simulink model "downlink_4c2t"  (Simulink 8.7)
settings: Solver=VariableStepDiscrete  StartTime=0.0  StopTime=DUC_LINEUP_param.endTime  RelTol=1e-3
PreLoadFcn:
  | % Run the setup script when the model is opened
  | setup_downlink_4c2t;
InitFcn:
  | % Run the setup script again just before the
  | % model is run, so that any updates made
  | % after opening are applied.
  | setup_downlink_4c2t;
  | 
  | %% DSPBuilder Start
  | alt_dspbuilder_update_model(bdroot)
  | %% DSPBuilder End
values from neighbouring files (symbols this model uses):
  LUTS_DPD_CLIP =     [downlink_4c2t_dpd_clip.mat]
  PulsExtention = 128    [setup_downlink_4c2t.m]
  StartAddress1 = Iter1_Param.BaseAddr + 3200    [setup_downlink_4c2t.m]
  StartAddress2 = StartAddress1+1024    [setup_downlink_4c2t.m]
  win = [w(1:PulsExtention) ones(1,Iter0_Param.pulseLen) w(PulsExtention+1:end)]    [setup_downlink_4c2t.m]
undefined symbols (not defined in the file or in its folder): AdvDSPBChannelOutDisplay, AdvDSPBDMemDisplay, dpoly, dspba_ChannelInVis, dspba_ChannelOutVis, dspba_internal_get_channel_ports, dspba_internal_get_demux_ports, DUC_LINEUP_param, evalAionMaskParam, iq_width, Iter0_Param, latency, primtype, REG, UseDontCare, value
undefined symbols (not defined in the file): cfr0_id, cfr_Params0, cfr_Params1, clock_rate, REG_dut_id_addr
libraries: DSPBAPrim x1438, DSPBAControl x77, DSPBAModelBus x71, DSPBABase x40, downlink_4c2t_foldingcfr_3firs_lib x26, DSPBAUtilities x8, downlink_4c2t_lib x4, downlink_4c2t_cordic_lib x2, downlink_4c2t_dpd_clipper x2, DSPBAFilters x2, DSPBAWaveformSynth x2, downlink_4c2t_lduc_lib x1
(part 11 of 17)

== system downlink_4c2t/DUT/Gain_dpd_input/Subsystem ==
  a : Inport
  v : Inport  Port=2
  c : Inport  Port=3
  dpd1_gain_val : Inport  Port=4
  dpd2_gain_val : Inport  Port=5
  ChannelIn : DSPBAPrim/ChannelIn  primtype=channelin  nInputs=dspba_internal_get_channel_ports(gcb)  nOutputs=dspba_internal_get_channel_ports(gcb)  omode=Inherit via internal rule  otype=sfix(16)  scale=2^-15  rndmethod=Unbiased  factor=1  satmethod=Symmetric  shift_vec=[0 1 2 -1]  value=1  inPortNames=['v'; 'c'; '0'; '1'; '2'; '3'; '4'; '5'; '6'; '7'; '8'; '9'; 'A'; 'B'; 'D'; 'E'; 'F'; 'G'; 'H'; 'I'; 'J'; 'K'; 'L'; 'M'; 'N'; 'O'; 'P'; 'Q'; 'R'; 'S'; 'T'; 'U'; 'W'; 'X'; 'Y'; 'Z']  outPortNames=['v'; 'c'; '0'; '1'; '2'; '3'; '4'; '5'; '6'; '7'; '8'; '9'; 'A'; 'B'; 'D'; 'E'; 'F'; 'G'; 'H'; 'I'; 'J'; 'K'; 'L'; 'M'; 'N'; 'O'; 'P'; 'Q'; 'R'; 'S'; 'T'; 'U'; 'W'; 'X'; 'Y'; 'Z']  dspbaimage=dspba_prim.jpg  text=fprintf('In');  style=Optimised  dataSignals=1  foldingEnabled=off  channels=1  sampleRate=200  packetBeginPresent=off  packetBeginEnabled=off  visibilities=dspba_ChannelInVis(gcb)  latencyCorrection=0  version=20141013
  ChannelOut : DSPBAPrim/ChannelOut  primtype=channelout  nInputs=dspba_internal_get_channel_ports(gcb)  nOutputs=dspba_internal_get_channel_ports(gcb)  omode=Inherit via internal rule  otype=sfix(16)  scale=2^-15  rndmethod=Unbiased  factor=1  satmethod=Symmetric  shift_vec=[0 1 2 -1]  value=1  inPortNames=['v'; 'c'; '0'; '1'; '2'; '3'; '4'; '5'; '6'; '7'; '8'; '9'; 'A'; 'B'; 'D'; 'E'; 'F'; 'G'; 'H'; 'I'; 'J'; 'K'; 'L'; 'M'; 'N'; 'O'; 'P'; 'Q'; 'R'; 'S'; 'T'; 'U'; 'W'; 'X'; 'Y'; 'Z']  outPortNames=['v'; 'c'; '0'; '1'; '2'; '3'; '4'; '5'; '6'; '7'; '8'; '9'; 'A'; 'B'; 'D'; 'E'; 'F'; 'G'; 'H'; 'I'; 'J'; 'K'; 'L'; 'M'; 'N'; 'O'; 'P'; 'Q'; 'R'; 'S'; 'T'; 'U'; 'W'; 'X'; 'Y'; 'Z']  dspbaimage=dspba_prim.jpg  text=fprintf('Out%s', AdvDSPBChannelOutDisplay(latency));  style=Optimised  dataSignals=1  foldingEnabled=off  channels=1  sampleRate=200  packetBeginPresent=off  packetBeginEnabled=off  visibilities=dspba_ChannelOutVis(gcb)  latency=4  latencyCorrection=0  version=20141013
  Demux : Demux
  GPIn1 : DSPBAPrim/GPIn  primtype=gpin  nInputs=evalAionMaskParam(gcb,'value',1)  nOutputs=evalAionMaskParam(gcb,'value',1)  omode=Inherit via internal rule  otype=sfix(16)  scale=2^-15  rndmethod=Unbiased  factor=1  satmethod=Symmetric  shift_vec=[0 1 2 -1]  value=1  inPortNames=[' ' ' ' ' ' ' ' ' ' ' ' ' ' ' ' ' ' ' ' ' ' ' ' ' ' ' ' ' ' ' ' ' ' ' ' ' ' ' ' ' ' ' ' ' ' ' ' ' ' ' ' ' ' ' ' ' ' ' ' ' ' ' ' ' ' ' ' ' ']'  outPortNames=[' ' ' ' ' ' ' ' ' ' ' ' ' ' ' ' ' ' ' ' ' ' ' ' ' ' ' ' ' ' ' ' ' ' ' ' ' ' ' ' ' ' ' ' ' ' ' ' ' ' ' ' ' ' ' ' ' ' ' ' ' ' ' ' ' ' ' ' ' ']'  dspbaimage=dspba_prim.jpg  text=fprintf('GPIn');  style=Optimised  visibilities=1024  latencyCorrection=0  version=20090407
  GPIn2 : DSPBAPrim/GPIn  primtype=gpin  nInputs=evalAionMaskParam(gcb,'value',1)  nOutputs=evalAionMaskParam(gcb,'value',1)  omode=Inherit via internal rule  otype=sfix(16)  scale=2^-15  rndmethod=Unbiased  factor=1  satmethod=Symmetric  shift_vec=[0 1 2 -1]  value=1  inPortNames=[' ' ' ' ' ' ' ' ' ' ' ' ' ' ' ' ' ' ' ' ' ' ' ' ' ' ' ' ' ' ' ' ' ' ' ' ' ' ' ' ' ' ' ' ' ' ' ' ' ' ' ' ' ' ' ' ' ' ' ' ' ' ' ' ' ' ' ' ' ']'  outPortNames=[' ' ' ' ' ' ' ' ' ' ' ' ' ' ' ' ' ' ' ' ' ' ' ' ' ' ' ' ' ' ' ' ' ' ' ' ' ' ' ' ' ' ' ' ' ' ' ' ' ' ' ' ' ' ' ' ' ' ' ' ' ' ' ' ' ' ' ' ' ']'  dspbaimage=dspba_prim.jpg  text=fprintf('GPIn');  style=Optimised  visibilities=1024  latencyCorrection=0  version=20090407
  LocalThreshold : DSPBABase/LocalThreshold  margin=DUC_LINEUP_param.ClockMargin  delayRegOrRAMThresholdBits=-1  MediumDualMemThresholdBits=-1  LargeDualMemThresholdBits=-1  hardMultiplierThresholdLuts=-1  complexMultKaratsuba=off  version=0
  Mult{,1..3} (4 alike) : DSPBAPrim/Mult  primtype=mult  nInputs=2  nOutputs=1  omode=Inherit via internal rule  otype=sfix(16)  scale=2^-15  rndmethod=Unbiased  factor=1  satmethod=Symmetric  shift_vec=[0 1 2 -1]  value=0  inPortNames=[' '; ' ';]  outPortNames=[' ']  dspbaimage=dspba_prim.jpg  text=fprintf('X');  style=Optimised  visibilities=8+2^18+2^19  floatPrecision=float32_m23  floatRounding=correct  advOptions=[]  version=20130115
  Mux : Mux
  SynthesisInfo : DSPBAPrim/SynthesisInfo  primtype=synthinfo  nInputs=0  nOutputs=0  omode=Inherit via internal rule  otype=sfix(16)  scale=2^-15  rndmethod=Truncate  factor=1  satmethod=Symmetric  shift_vec=[0 1 2 -1]  value=99  inPortNames=[' '; ' ';]  outPortNames=[' ']  dspbaimage=dspba_prim_ctrl.jpg  text=fprintf('Style=%s', style);  style=Scheduled  visibilities=2^15+2^17+2^18+2^19  constraintInUse=off  constraintRelation=>  constraintLimit=8  bitAccurate=off  version=20150220
  gain_v_out : Outport
  gain_c_out : Outport  Port=2
  gain_real_out : Outport  Port=3
  wires:
  GPIn1/1 -> Mult1/2, Mult/2
  ChannelOut/2 -> gain_c_out/1
  ChannelOut/1 -> gain_v_out/1
  dpd2_gain_val/1 -> GPIn2/1
  dpd1_gain_val/1 -> GPIn1/1
  ChannelOut/3 -> gain_real_out/1
  v/1 -> ChannelIn/1
  c/1 -> ChannelIn/2
  a/1 -> ChannelIn/3
  ChannelIn/1 -> ChannelOut/1
  ChannelIn/2 -> ChannelOut/2
  ChannelIn/3 -> Demux/1
  Demux/1 -> Mult/1
  Demux/2 -> Mult1/1
  Demux/3 -> Mult2/1
  GPIn2/1 -> Mult3/2, Mult2/2
  Demux/4 -> Mult3/1
  Mult/1 -> Mux/1
  Mult1/1 -> Mux/2
  Mult2/1 -> Mux/3
  Mult3/1 -> Mux/4
  Mux/1 -> ChannelOut/3

== system downlink_4c2t/DUT/Gain_duc_input/gain ==
  a : Inport
  v : Inport  Port=2
  c : Inport  Port=3
  carr1_gain_val : Inport  Port=4
  carr2_gain_val : Inport  Port=5
  carr3_gain_val : Inport  Port=6
  carr4_gain_val : Inport  Port=7
  carr5_gain_val : Inport  Port=8
  carr6_gain_val : Inport  Port=9
  carr7_gain_val : Inport  Port=10
  carr8_gain_val : Inport  Port=11
  BitExtract : DSPBAPrim/BitExtract  primtype=bitextract  nInputs=1  nOutputs=1  omode=Specify via dialog  otype=ufix(4)  scale=2^-0  rndmethod=Unbiased  factor=1  satmethod=Symmetric  shift_vec=[0 1 2 -1]  value=1  inPortNames=[' '; ' ';]  outPortNames=[' ']  dspbaimage=dspba_prim.jpg  text=fprintf('..%d', value);  style=Optimised  visibilities=8+1024  version=20090407
  ChannelIn : DSPBAPrim/ChannelIn  primtype=channelin  nInputs=dspba_internal_get_channel_ports(gcb)  nOutputs=dspba_internal_get_channel_ports(gcb)  omode=Inherit via internal rule  otype=sfix(16)  scale=2^-15  rndmethod=Unbiased  factor=1  satmethod=Symmetric  shift_vec=[0 1 2 -1]  value=1  inPortNames=['v'; 'c'; '0'; '1'; '2'; '3'; '4'; '5'; '6'; '7'; '8'; '9'; 'A'; 'B'; 'D'; 'E'; 'F'; 'G'; 'H'; 'I'; 'J'; 'K'; 'L'; 'M'; 'N'; 'O'; 'P'; 'Q'; 'R'; 'S'; 'T'; 'U'; 'W'; 'X'; 'Y'; 'Z']  outPortNames=['v'; 'c'; '0'; '1'; '2'; '3'; '4'; '5'; '6'; '7'; '8'; '9'; 'A'; 'B'; 'D'; 'E'; 'F'; 'G'; 'H'; 'I'; 'J'; 'K'; 'L'; 'M'; 'N'; 'O'; 'P'; 'Q'; 'R'; 'S'; 'T'; 'U'; 'W'; 'X'; 'Y'; 'Z']  dspbaimage=dspba_prim.jpg  text=fprintf('In');  style=Optimised  dataSignals=1  foldingEnabled=off  channels=1  sampleRate=200  packetBeginPresent=off  packetBeginEnabled=off  visibilities=dspba_ChannelInVis(gcb)  latencyCorrection=0  version=20141013
  ChannelOut : DSPBAPrim/ChannelOut  primtype=channelout  nInputs=dspba_internal_get_channel_ports(gcb)  nOutputs=dspba_internal_get_channel_ports(gcb)  omode=Inherit via internal rule  otype=sfix(16)  scale=2^-15  rndmethod=Unbiased  factor=1  satmethod=Symmetric  shift_vec=[0 1 2 -1]  value=1  inPortNames=['v'; 'c'; '0'; '1'; '2'; '3'; '4'; '5'; '6'; '7'; '8'; '9'; 'A'; 'B'; 'D'; 'E'; 'F'; 'G'; 'H'; 'I'; 'J'; 'K'; 'L'; 'M'; 'N'; 'O'; 'P'; 'Q'; 'R'; 'S'; 'T'; 'U'; 'W'; 'X'; 'Y'; 'Z']  outPortNames=['v'; 'c'; '0'; '1'; '2'; '3'; '4'; '5'; '6'; '7'; '8'; '9'; 'A'; 'B'; 'D'; 'E'; 'F'; 'G'; 'H'; 'I'; 'J'; 'K'; 'L'; 'M'; 'N'; 'O'; 'P'; 'Q'; 'R'; 'S'; 'T'; 'U'; 'W'; 'X'; 'Y'; 'Z']  dspbaimage=dspba_prim.jpg  text=fprintf('Out%s', AdvDSPBChannelOutDisplay(latency));  style=Optimised  dataSignals=1  foldingEnabled=off  channels=1  sampleRate=200  packetBeginPresent=off  packetBeginEnabled=off  visibilities=dspba_ChannelOutVis(gcb)  latency=5  latencyCorrection=0  version=20141013
  GPIn{1..8} (8 alike) : DSPBAPrim/GPIn  primtype=gpin  nInputs=evalAionMaskParam(gcb,'value',1)  nOutputs=evalAionMaskParam(gcb,'value',1)  omode=Inherit via internal rule  otype=sfix(16)  scale=2^-15  rndmethod=Unbiased  factor=1  satmethod=Symmetric  shift_vec=[0 1 2 -1]  value=1  inPortNames=[' ' ' ' ' ' ' ' ' ' ' ' ' ' ' ' ' ' ' ' ' ' ' ' ' ' ' ' ' ' ' ' ' ' ' ' ' ' ' ' ' ' ' ' ' ' ' ' ' ' ' ' ' ' ' ' ' ' ' ' ' ' ' ' ' ' ' ' ' ']'  outPortNames=[' ' ' ' ' ' ' ' ' ' ' ' ' ' ' ' ' ' ' ' ' ' ' ' ' ' ' ' ' ' ' ' ' ' ' ' ' ' ' ' ' ' ' ' ' ' ' ' ' ' ' ' ' ' ' ' ' ' ' ' ' ' ' ' ' ' ' ' ' ']'  dspbaimage=dspba_prim.jpg  text=fprintf('GPIn');  style=Optimised  visibilities=1024  latencyCorrection=0  version=20090407
  LocalThreshold : DSPBABase/LocalThreshold  margin=DUC_LINEUP_param.ClockMargin  delayRegOrRAMThresholdBits=-1  MediumDualMemThresholdBits=-1  LargeDualMemThresholdBits=-1  hardMultiplierThresholdLuts=-1  complexMultKaratsuba=off  version=0
  Mult : DSPBAPrim/Mult  primtype=mult  nInputs=2  nOutputs=1  omode=Inherit via internal rule  otype=sfix(16)  scale=2^-15  rndmethod=Unbiased  factor=1  satmethod=Symmetric  shift_vec=[0 1 2 -1]  value=0  inPortNames=[' '; ' ';]  outPortNames=[' ']  dspbaimage=dspba_prim.jpg  text=fprintf('X');  style=Optimised  visibilities=8+2^18+2^19  floatPrecision=float32_m23  floatRounding=correct  advOptions=[]  version=20130115
  Mux : DSPBAPrim/Mux  primtype=mux  nInputs=evalAionMaskParam(gcb,'value',1)+1  nOutputs=1  omode=Inherit via internal rule  otype=sfix(16)  scale=2^-15  rndmethod=Unbiased  factor=1  satmethod=Symmetric  shift_vec=[0 1 2 -1]  value=8  inPortNames=['s '; 'd0'; 'd1'; 'd2'; 'd3'; 'd4'; 'd5'; 'd6'; 'd7'; 'd8'; 'd9';]  outPortNames=[' ']  dspbaimage=dspba_prim.jpg  text=fprintf('%s', primtype);  style=Optimised  visibilities=1032  version=20131025
  SynthesisInfo : DSPBAPrim/SynthesisInfo  primtype=synthinfo  nInputs=0  nOutputs=0  omode=Inherit via internal rule  otype=sfix(16)  scale=2^-15  rndmethod=Truncate  factor=1  satmethod=Symmetric  shift_vec=[0 1 2 -1]  value=99  inPortNames=[' '; ' ';]  outPortNames=[' ']  dspbaimage=dspba_prim_ctrl.jpg  text=fprintf('Style=%s', style);  style=Scheduled  visibilities=2^15+2^17+2^18+2^19  constraintInUse=off  constraintRelation=>  constraintLimit=8  bitAccurate=off  version=20150220
  gain_v_out : Outport
  gain_c_out : Outport  Port=2
  gain_real_out : Outport  Port=3
  wires:
  carr3_gain_val/1 -> GPIn3/1
  BitExtract/1 -> Mux/1
  Mult/1 -> ChannelOut/3
  ChannelIn/2 -> ChannelOut/2, BitExtract/1
  ChannelIn/1 -> ChannelOut/1
  a/1 -> ChannelIn/3
  c/1 -> ChannelIn/2
  v/1 -> ChannelIn/1
  Mux/1 -> Mult/2
  ChannelOut/3 -> gain_real_out/1
  carr8_gain_val/1 -> GPIn8/1
  carr1_gain_val/1 -> GPIn1/1
  carr4_gain_val/1 -> GPIn4/1
  carr5_gain_val/1 -> GPIn5/1
  carr6_gain_val/1 -> GPIn6/1
  carr2_gain_val/1 -> GPIn2/1
  carr7_gain_val/1 -> GPIn7/1
  ChannelIn/3 -> Mult/1
  ChannelOut/1 -> gain_v_out/1
  ChannelOut/2 -> gain_c_out/1
  GPIn1/1 -> Mux/2
  GPIn2/1 -> Mux/3
  GPIn3/1 -> Mux/4
  GPIn4/1 -> Mux/5
  GPIn5/1 -> Mux/6
  GPIn6/1 -> Mux/7
  GPIn7/1 -> Mux/8
  GPIn8/1 -> Mux/9

== system downlink_4c2t/DUT/Gain_summer/Subsystem ==
  a : Inport
  v : Inport  Port=2
  c : Inport  Port=3
  ant1_gain_val : Inport  Port=4
  ant2_gain_val : Inport  Port=5
  BitExtract : DSPBAPrim/BitExtract  primtype=bitextract  nInputs=1  nOutputs=1  omode=Specify via dialog  otype=ufix(4)  scale=2^-0  rndmethod=Unbiased  factor=1  satmethod=Symmetric  shift_vec=[0 1 2 -1]  value=1  inPortNames=[' '; ' ';]  outPortNames=[' ']  dspbaimage=dspba_prim.jpg  text=fprintf('..%d', value);  style=Optimised  visibilities=8+1024  version=20090407
  ChannelIn : DSPBAPrim/ChannelIn  primtype=channelin  nInputs=dspba_internal_get_channel_ports(gcb)  nOutputs=dspba_internal_get_channel_ports(gcb)  omode=Inherit via internal rule  otype=sfix(16)  scale=2^-15  rndmethod=Unbiased  factor=1  satmethod=Symmetric  shift_vec=[0 1 2 -1]  value=1  inPortNames=['v'; 'c'; '0'; '1'; '2'; '3'; '4'; '5'; '6'; '7'; '8'; '9'; 'A'; 'B'; 'D'; 'E'; 'F'; 'G'; 'H'; 'I'; 'J'; 'K'; 'L'; 'M'; 'N'; 'O'; 'P'; 'Q'; 'R'; 'S'; 'T'; 'U'; 'W'; 'X'; 'Y'; 'Z']  outPortNames=['v'; 'c'; '0'; '1'; '2'; '3'; '4'; '5'; '6'; '7'; '8'; '9'; 'A'; 'B'; 'D'; 'E'; 'F'; 'G'; 'H'; 'I'; 'J'; 'K'; 'L'; 'M'; 'N'; 'O'; 'P'; 'Q'; 'R'; 'S'; 'T'; 'U'; 'W'; 'X'; 'Y'; 'Z']  dspbaimage=dspba_prim.jpg  text=fprintf('In');  style=Optimised  dataSignals=1  foldingEnabled=off  channels=1  sampleRate=200  packetBeginPresent=off  packetBeginEnabled=off  visibilities=dspba_ChannelInVis(gcb)  latencyCorrection=0  version=20141013
  ChannelOut : DSPBAPrim/ChannelOut  primtype=channelout  nInputs=dspba_internal_get_channel_ports(gcb)  nOutputs=dspba_internal_get_channel_ports(gcb)  omode=Inherit via internal rule  otype=sfix(16)  scale=2^-15  rndmethod=Unbiased  factor=1  satmethod=Symmetric  shift_vec=[0 1 2 -1]  value=1  inPortNames=['v'; 'c'; '0'; '1'; '2'; '3'; '4'; '5'; '6'; '7'; '8'; '9'; 'A'; 'B'; 'D'; 'E'; 'F'; 'G'; 'H'; 'I'; 'J'; 'K'; 'L'; 'M'; 'N'; 'O'; 'P'; 'Q'; 'R'; 'S'; 'T'; 'U'; 'W'; 'X'; 'Y'; 'Z']  outPortNames=['v'; 'c'; '0'; '1'; '2'; '3'; '4'; '5'; '6'; '7'; '8'; '9'; 'A'; 'B'; 'D'; 'E'; 'F'; 'G'; 'H'; 'I'; 'J'; 'K'; 'L'; 'M'; 'N'; 'O'; 'P'; 'Q'; 'R'; 'S'; 'T'; 'U'; 'W'; 'X'; 'Y'; 'Z']  dspbaimage=dspba_prim.jpg  text=fprintf('Out%s', AdvDSPBChannelOutDisplay(latency));  style=Optimised  dataSignals=1  foldingEnabled=off  channels=1  sampleRate=200  packetBeginPresent=off  packetBeginEnabled=off  visibilities=dspba_ChannelOutVis(gcb)  latency=4  latencyCorrection=0  version=20141013
  GPIn1 : DSPBAPrim/GPIn  primtype=gpin  nInputs=evalAionMaskParam(gcb,'value',1)  nOutputs=evalAionMaskParam(gcb,'value',1)  omode=Inherit via internal rule  otype=sfix(16)  scale=2^-15  rndmethod=Unbiased  factor=1  satmethod=Symmetric  shift_vec=[0 1 2 -1]  value=1  inPortNames=[' ' ' ' ' ' ' ' ' ' ' ' ' ' ' ' ' ' ' ' ' ' ' ' ' ' ' ' ' ' ' ' ' ' ' ' ' ' ' ' ' ' ' ' ' ' ' ' ' ' ' ' ' ' ' ' ' ' ' ' ' ' ' ' ' ' ' ' ' ']'  outPortNames=[' ' ' ' ' ' ' ' ' ' ' ' ' ' ' ' ' ' ' ' ' ' ' ' ' ' ' ' ' ' ' ' ' ' ' ' ' ' ' ' ' ' ' ' ' ' ' ' ' ' ' ' ' ' ' ' ' ' ' ' ' ' ' ' ' ' ' ' ' ']'  dspbaimage=dspba_prim.jpg  text=fprintf('GPIn');  style=Optimised  visibilities=1024  latencyCorrection=0  version=20090407
  GPIn2 : DSPBAPrim/GPIn  primtype=gpin  nInputs=evalAionMaskParam(gcb,'value',1)  nOutputs=evalAionMaskParam(gcb,'value',1)  omode=Inherit via internal rule  otype=sfix(16)  scale=2^-15  rndmethod=Unbiased  factor=1  satmethod=Symmetric  shift_vec=[0 1 2 -1]  value=1  inPortNames=[' ' ' ' ' ' ' ' ' ' ' ' ' ' ' ' ' ' ' ' ' ' ' ' ' ' ' ' ' ' ' ' ' ' ' ' ' ' ' ' ' ' ' ' ' ' ' ' ' ' ' ' ' ' ' ' ' ' ' ' ' ' ' ' ' ' ' ' ' ']'  outPortNames=[' ' ' ' ' ' ' ' ' ' ' ' ' ' ' ' ' ' ' ' ' ' ' ' ' ' ' ' ' ' ' ' ' ' ' ' ' ' ' ' ' ' ' ' ' ' ' ' ' ' ' ' ' ' ' ' ' ' ' ' ' ' ' ' ' ' ' ' ' ']'  dspbaimage=dspba_prim.jpg  text=fprintf('GPIn');  style=Optimised  visibilities=1024  latencyCorrection=0  version=20090407
  LocalThreshold : DSPBABase/LocalThreshold  margin=DUC_LINEUP_param.ClockMargin  delayRegOrRAMThresholdBits=-1  MediumDualMemThresholdBits=-1  LargeDualMemThresholdBits=-1  hardMultiplierThresholdLuts=-1  complexMultKaratsuba=off  version=0
  Mult : DSPBAPrim/Mult  primtype=mult  nInputs=2  nOutputs=1  omode=Inherit via internal rule  otype=sfix(16)  scale=2^-15  rndmethod=Unbiased  factor=1  satmethod=Symmetric  shift_vec=[0 1 2 -1]  value=0  inPortNames=[' '; ' ';]  outPortNames=[' ']  dspbaimage=dspba_prim.jpg  text=fprintf('X');  style=Optimised  visibilities=8+2^18+2^19  floatPrecision=float32_m23  floatRounding=correct  advOptions=[]  version=20130115
  Mux : DSPBAPrim/Mux  primtype=mux  nInputs=evalAionMaskParam(gcb,'value',1)+1  nOutputs=1  omode=Inherit via internal rule  otype=sfix(16)  scale=2^-15  rndmethod=Unbiased  factor=1  satmethod=Symmetric  shift_vec=[0 1 2 -1]  value=2  inPortNames=['s '; 'd0'; 'd1'; 'd2'; 'd3'; 'd4'; 'd5'; 'd6'; 'd7'; 'd8'; 'd9';]  outPortNames=[' ']  dspbaimage=dspba_prim.jpg  text=fprintf('%s', primtype);  style=Optimised  visibilities=1032  version=20131025
  SynthesisInfo : DSPBAPrim/SynthesisInfo  primtype=synthinfo  nInputs=0  nOutputs=0  omode=Inherit via internal rule  otype=sfix(16)  scale=2^-15  rndmethod=Truncate  factor=1  satmethod=Symmetric  shift_vec=[0 1 2 -1]  value=99  inPortNames=[' '; ' ';]  outPortNames=[' ']  dspbaimage=dspba_prim_ctrl.jpg  text=fprintf('Style=%s', style);  style=Scheduled  visibilities=2^15+2^17+2^18+2^19  constraintInUse=off  constraintRelation=>  constraintLimit=6  bitAccurate=off  version=20150220
  gain_v_out : Outport
  gain_c_out : Outport  Port=2
  gain_real_out : Outport  Port=3
  wires:
  GPIn2/1 -> Mux/3
  GPIn1/1 -> Mux/2
  ChannelOut/2 -> gain_c_out/1
  ChannelOut/1 -> gain_v_out/1
  ChannelIn/3 -> Mult/1
  ant2_gain_val/1 -> GPIn2/1
  ant1_gain_val/1 -> GPIn1/1
  ChannelOut/3 -> gain_real_out/1
  Mux/1 -> Mult/2
  v/1 -> ChannelIn/1
  c/1 -> ChannelIn/2
  a/1 -> ChannelIn/3
  ChannelIn/1 -> ChannelOut/1
  ChannelIn/2 -> ChannelOut/2, BitExtract/1
  Mult/1 -> ChannelOut/3
  BitExtract/1 -> Mux/1

== system downlink_4c2t/DUT/LDUC/Mixer_Summer ==
  In_a : Inport
  In_V : Inport  Port=2
  In_C : Inport  Port=3
  In_sync_pulse : Inport  Port=4
  sum_shift : Inport  Port=5
  COMPLEX_MIXER : Subsystem
  PipeReg_2in : downlink_4c2t_foldingcfr_3firs_lib/PipeReg_2in  NPipe=2  Clock_Margin=DUC_LINEUP_param.ClockMargin
      link override ChannelOut: value=2  packetBeginEnabled=off  latency=2
  PipeReg_2in1 : downlink_4c2t_foldingcfr_3firs_lib/PipeReg_2in  NPipe=2  Clock_Margin=DUC_LINEUP_param.ClockMargin
      link override ChannelOut: value=2  packetBeginEnabled=off  latency=2
  SUMMER : Subsystem
  Out_q : Outport
  Out_V : Outport  Port=2
  Out_C : Outport  Port=3
  wires:
  SUMMER/2(q_v) -> Out_V/1
  In_V/1 -> COMPLEX_MIXER/2(v)
  In_C/1 -> COMPLEX_MIXER/3(c)
  SUMMER/1(q) -> Out_q/1
  In_a/1 -> COMPLEX_MIXER/1(a)
  SUMMER/3(q_c) -> Out_C/1
  In_sync_pulse/1 -> COMPLEX_MIXER/4(sync_pulse)
  COMPLEX_MIXER/1(out_I) -> PipeReg_2in/1
  COMPLEX_MIXER/2(out_q) -> PipeReg_2in/2
  COMPLEX_MIXER/4(q_c) -> PipeReg_2in/4
  COMPLEX_MIXER/3(q_v) -> PipeReg_2in/3
  PipeReg_2in/4 -> PipeReg_2in1/4
  PipeReg_2in/1 -> PipeReg_2in1/1
  PipeReg_2in/2 -> PipeReg_2in1/2
  PipeReg_2in/3 -> PipeReg_2in1/3
  PipeReg_2in1/1 -> SUMMER/1(a)
  PipeReg_2in1/2 -> SUMMER/2(a1)
  PipeReg_2in1/3 -> SUMMER/3(v)
  PipeReg_2in1/4 -> SUMMER/4(c)
  sum_shift/1 -> SUMMER/5(sum_shift)

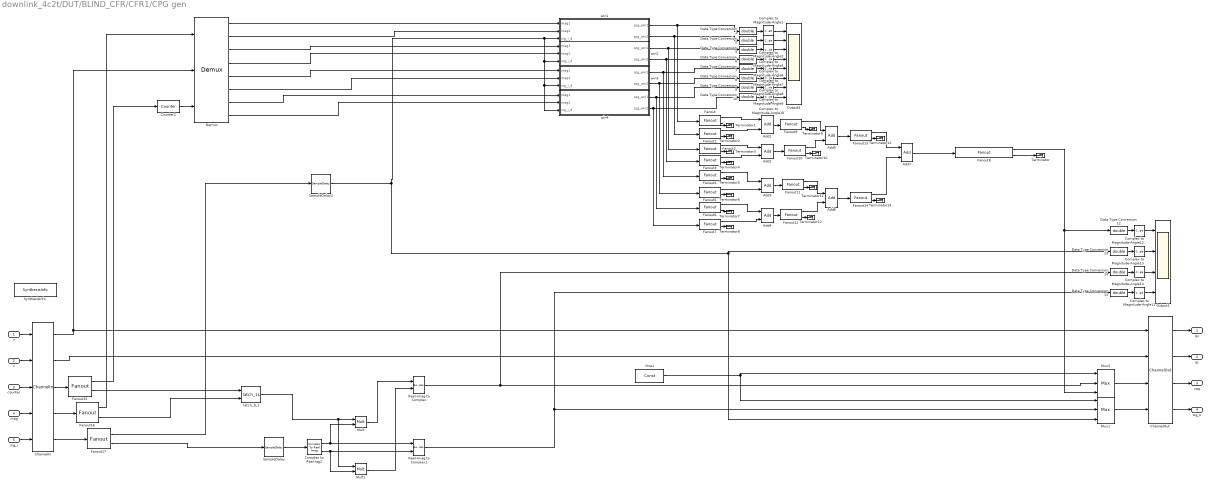
== system downlink_4c2t/DUT/BLIND_CFR/CFR1/CPG gen ==
  v : Inport
  c : Inport  Port=2
  counter : Inport  Port=3
  mag : Inport  Port=4
  sig_i : Inport  Port=5
  Add{1..7} (7 alike) : DSPBAPrim/Add  primtype=add  nInputs=evalAionMaskParam(gcb,'value',1)  nOutputs=1  omode=Inherit via internal rule with word growth  otype=sfix(16)  scale=2^-15  rndmethod=Unbiased  factor=1  satmethod=Symmetric  shift_vec=[0 1 2 -1]  value=2  inPortNames=[' '; ' ';]  outPortNames=[' ']  dspbaimage=dspba_prim.jpg  text=fprintf('+');  style=Optimised  visibilities=1032+2^17+2^18+2^19  genFPC=off  floatRounding=correct  advOptions=[]  version=20130821
  ChannelIn : DSPBAPrim/ChannelIn  primtype=channelin  nInputs=dspba_internal_get_channel_ports(gcb)  nOutputs=dspba_internal_get_channel_ports(gcb)  omode=Inherit via internal rule  otype=sfix(16)  scale=2^-15  rndmethod=Unbiased  factor=1  satmethod=Symmetric  shift_vec=[0 1 2 -1]  value=3  inPortNames=['v'; 'c'; '0'; '1'; '2'; '3'; '4'; '5'; '6'; '7'; '8'; '9'; 'A'; 'B'; 'D'; 'E'; 'F'; 'G'; 'H'; 'I'; 'J'; 'K'; 'L'; 'M'; 'N'; 'O'; 'P'; 'Q'; 'R'; 'S'; 'T'; 'U'; 'W'; 'X'; 'Y'; 'Z']  outPortNames=['v'; 'c'; '0'; '1'; '2'; '3'; '4'; '5'; '6'; '7'; '8'; '9'; 'A'; 'B'; 'D'; 'E'; 'F'; 'G'; 'H'; 'I'; 'J'; 'K'; 'L'; 'M'; 'N'; 'O'; 'P'; 'Q'; 'R'; 'S'; 'T'; 'U'; 'W'; 'X'; 'Y'; 'Z']  dspbaimage=dspba_prim.jpg  text=fprintf('In');  style=Optimised  dataSignals=3  foldingEnabled=off  channels=1  sampleRate=200  packetBeginPresent=off  packetBeginEnabled=off  visibilities=dspba_ChannelInVis(gcb)  latencyCorrection=0  version=20141013
  ChannelOut : DSPBAPrim/ChannelOut  primtype=channelout  nInputs=dspba_internal_get_channel_ports(gcb)  nOutputs=dspba_internal_get_channel_ports(gcb)  omode=Inherit via internal rule  otype=sfix(16)  scale=2^-15  rndmethod=Unbiased  factor=1  satmethod=Symmetric  shift_vec=[0 1 2 -1]  value=2  inPortNames=['v'; 'c'; '0'; '1'; '2'; '3'; '4'; '5'; '6'; '7'; '8'; '9'; 'A'; 'B'; 'D'; 'E'; 'F'; 'G'; 'H'; 'I'; 'J'; 'K'; 'L'; 'M'; 'N'; 'O'; 'P'; 'Q'; 'R'; 'S'; 'T'; 'U'; 'W'; 'X'; 'Y'; 'Z']  outPortNames=['v'; 'c'; '0'; '1'; '2'; '3'; '4'; '5'; '6'; '7'; '8'; '9'; 'A'; 'B'; 'D'; 'E'; 'F'; 'G'; 'H'; 'I'; 'J'; 'K'; 'L'; 'M'; 'N'; 'O'; 'P'; 'Q'; 'R'; 'S'; 'T'; 'U'; 'W'; 'X'; 'Y'; 'Z']  dspbaimage=dspba_prim.jpg  text=fprintf('Out%s', AdvDSPBChannelOutDisplay(latency));  style=Optimised  dataSignals=2  foldingEnabled=off  channels=1  sampleRate=200  packetBeginPresent=off  packetBeginEnabled=off  visibilities=dspba_ChannelOutVis(gcb)  latency=28  latencyCorrection=0  version=20141013
  Complex to Magnitude-Angle{1..2,5..14} (12 alike) : ComplexToMagnitudeAngle  Output=Magnitude
  Complex to Real-Iag2 : ComplexToRealImag
  Counter2 : DSPBAPrim/Counter  primtype=counter  nInputs=1  nOutputs=1  omode=Inherit via internal rule  otype=ufix(16)  scale=2^-0  rndmethod=Unbiased  factor=1  satmethod=Symmetric  shift_vec=[0 1 2 -1]  value=[0 8 1]  inPortNames=[' '; ' ';]  outPortNames=[' ']  dspbaimage=dspba_prim.jpg  text=fprintf('counter\n[%d %d %d]', value(1), value(2), value(3));  style=Optimised  visibilities=8 + 1024  version=20090407
  Data Type Conversion{1..3,6..14} (12 alike) : DataTypeConversion  OutDataTypeStr=double
  Demux : DSPBAPrim/Demux  primtype=demux  nInputs=3  nOutputs=dspba_internal_get_demux_ports(gcb)  omode=Inherit via internal rule  otype=sfix(16)  scale=2^-15  rndmethod=Unbiased  factor=1  satmethod=Symmetric  shift_vec=[0 1 2 3 4 5 6 7]  value=8  inPortNames=['q'; 'v'; 'c']  outPortNames=['c0'; 'c1']  dspbaimage=dspba_prim.jpg  text=fprintf('demux');  style=Optimised  visibilities=1536  version=20100120
  Fanout{,1..17} (18 alike) : DSPBAPrim/Fanout  primtype=fanout  nInputs=1  nOutputs=evalAionMaskParam(gcb,'value',1)  omode=Inherit via internal rule  otype=sfix(16)  scale=2^-15  rndmethod=Unbiased  factor=1  satmethod=Symmetric  shift_vec=[0 1 2 -1]  value=2  inPortNames=[' '; ' ';]  outPortNames=[' ']  dspbaimage=dspba_prim.jpg  text=fprintf('fanout')  style=Optimised  visibilities=2^10+2^18  version=20150501  uninit=off
  Mult : DSPBAPrim/Mult  primtype=mult  nInputs=2  nOutputs=1  omode=Inherit via internal rule  otype=sfix(16)  scale=2^-15  rndmethod=Unbiased  factor=1  satmethod=Symmetric  shift_vec=[0 1 2 -1]  value=0  inPortNames=[' '; ' ';]  outPortNames=[' ']  dspbaimage=dspba_prim.jpg  text=fprintf('X');  style=Optimised  visibilities=8+2^18+2^19  floatPrecision=float32_m23  floatRounding=correct  advOptions=[]  version=20130115
  Mult1 : DSPBAPrim/Mult  primtype=mult  nInputs=2  nOutputs=1  omode=Inherit via internal rule  otype=sfix(16)  scale=2^-15  rndmethod=Unbiased  factor=1  satmethod=Symmetric  shift_vec=[0 1 2 -1]  value=0  inPortNames=[' '; ' ';]  outPortNames=[' ']  dspbaimage=dspba_prim.jpg  text=fprintf('X');  style=Optimised  visibilities=8+2^18+2^19  floatPrecision=float32_m23  floatRounding=correct  advOptions=[]  version=20130115
  Mux1 : DSPBAPrim/Mux  primtype=mux  nInputs=evalAionMaskParam(gcb,'value',1)+1  nOutputs=1  omode=Inherit via internal rule  otype=sfix(16)  scale=2^-15  rndmethod=Unbiased  factor=1  satmethod=Symmetric  shift_vec=[0 1 2 -1]  value=2  inPortNames=['s'; 'd0'; 'd1'; 'd2'; 'd3'; 'd4'; 'd5'; 'd6'; 'd7'; 'd8'; 'd9';]  outPortNames=[' ']  dspbaimage=dspba_prim.jpg  text=fprintf('%s', primtype);  style=Optimised  visibilities=1032  version=20131025
  Mux3 : DSPBAPrim/Mux  primtype=mux  nInputs=evalAionMaskParam(gcb,'value',1)+1  nOutputs=1  omode=Inherit via internal rule  otype=sfix(16)  scale=2^-15  rndmethod=Unbiased  factor=1  satmethod=Symmetric  shift_vec=[0 1 2 -1]  value=2  inPortNames=['s'; 'd0'; 'd1'; 'd2'; 'd3'; 'd4'; 'd5'; 'd6'; 'd7'; 'd8'; 'd9';]  outPortNames=[' ']  dspbaimage=dspba_prim.jpg  text=fprintf('%s', primtype);  style=Optimised  visibilities=1032  version=20131025
  One1 : DSPBAPrim/Const  primtype=const  nInputs=0  nOutputs=1  omode=boolean  otype=uint(1)  scale=2^0  rndmethod=Unbiased  factor=1  satmethod=Symmetric  shift_vec=[0 1 2 -1]  value=win_enable  inPortNames=['+'; '+';]  outPortNames=[' ']  dspbaimage=dspba_prim.jpg  text=fprintf('%s', num2str(value));  style=Optimised  visibilities=8 + 1024  floatPrecision=float32_m23  version=20120820
  Output1 : Scope  NumInputPorts=4
  Output5 : Scope  NumInputPorts=8
  Real-Imag to Complex : RealImagToComplex
  Real-Imag to Complex1 : RealImagToComplex
  SampleDelay : DSPBAPrim/SampleDelay  primtype=sampdelay  nInputs=1  nOutputs=1  omode=Inherit via internal rule  otype=uint(16)  scale=2^-0  rndmethod=Unbiased  factor=1  satmethod=Symmetric  shift_vec=[0 1 2 -1]  value=Iter0_Param.pulseLen  inPortNames=[' '; ' ';]  outPortNames=[' ']  dspbaimage=dspba_prim.jpg  text=dpoly(1, eye(1,value+1), 'z')  style=Optimised  visibilities=8 + 1024  flexible=off  slackgroup=0  augmented=0  version=20090407  advOptions=[]
  SampleDelay2 : DSPBAPrim/SampleDelay  primtype=sampdelay  nInputs=1  nOutputs=1  omode=Inherit via internal rule  otype=uint(16)  scale=2^-0  rndmethod=Unbiased  factor=1  satmethod=Symmetric  shift_vec=[0 1 2 -1]  value=Iter0_Param.pulseLen + PulsExtention  inPortNames=[' '; ' ';]  outPortNames=[' ']  dspbaimage=dspba_prim.jpg  text=dpoly(1, eye(1,value+1), 'z')  style=Optimised  visibilities=8 + 1024  flexible=off  slackgroup=0  augmented=0  version=20090407  advOptions=[]
  SynthesisInfo : DSPBAPrim/SynthesisInfo  primtype=synthinfo  nInputs=0  nOutputs=0  omode=Inherit via internal rule  otype=sfix(16)  scale=2^-15  rndmethod=Truncate  factor=1  satmethod=Symmetric  shift_vec=[0 1 2 -1]  value=99  inPortNames=[' '; ' ';]  outPortNames=[' ']  dspbaimage=dspba_prim.jpg  text=fprintf('Style=%s', style);  style=Scheduled  visibilities=32768  constraintInUse=off  constraintRelation=>  constraintLimit=50  bitAccurate=off  version=20150220
  Terminator{,1..14} (15 alike) : Terminator
  latch_1L1 : DSPBAControl/latch_1L
  win1 : Subsystem
  win2 : Subsystem
  win3 : Subsystem
  win4 : Subsystem
  qv : Outport
  qc : Outport  Port=2
  cpg : Outport  Port=3
  sig_o : Outport  Port=4
  wires:
  Mult/1 -> Real-Imag to Complex/1
  Mult1/1 -> Real-Imag to Complex/2
  Complex to Real-Iag2/2 -> Mult1/2, Real-Imag to Complex1/2
  v/1 -> ChannelIn/1
  c/1 -> ChannelIn/2
  ChannelIn/2 -> ChannelOut/2
  Real-Imag to Complex/1 -> Data Type Conversion14/1, Mux3/2
  ChannelOut/1 -> qv/1
  ChannelOut/2 -> qc/1
  counter/1 -> ChannelIn/3
  mag/1 -> ChannelIn/4
  ChannelOut/3 -> cpg/1
  ChannelOut/4 -> sig_o/1
  Complex to Real-Iag2/1 -> Mult/2, Real-Imag to Complex1/1
  Real-Imag to Complex1/1 -> Mux1/2, Data Type Conversion11/1
  sig_i/1 -> ChannelIn/5
  latch_1L1/1 -> Mult1/1, Mult/1
  ChannelIn/1 -> Demux/2, ChannelOut/1
  SampleDelay/1 -> Complex to Real-Iag2/1
  Counter2/1 -> Demux/3
  Data Type Conversion1/1 -> Complex to Magnitude-Angle1/1
  Complex to Magnitude-Angle1/1 -> Output5/1
  Data Type Conversion2/1 -> Complex to Magnitude-Angle2/1
  Complex to Magnitude-Angle2/1 -> Output5/2
  Demux/1 -> win1/1(mag1)
  Demux/2 -> win1/2(mag2)
  SampleDelay2/1 -> win1/3(sig_i_d), win2/3(sig_i_d), win4/3(sig_i_d), win3/3(sig_i_d), Mux1/3, Data Type Conversion13/1
  win1/1(cpg_win1) -> Data Type Conversion1/1, Fanout/1
  win1/2(cpg_win2) -> Fanout1/1, Data Type Conversion2/1
  Demux/3 -> win2/1(mag1)
  Demux/4 -> win2/2(mag2)
  Data Type Conversion3/1 -> Complex to Magnitude-Angle5/1
  Complex to Magnitude-Angle5/1 -> Output5/3
  Data Type Conversion6/1 -> Complex to Magnitude-Angle6/1
  Complex to Magnitude-Angle6/1 -> Output5/4
  Data Type Conversion7/1 -> Complex to Magnitude-Angle7/1
  Complex to Magnitude-Angle7/1 -> Output5/5
  Data Type Conversion8/1 -> Complex to Magnitude-Angle8/1
  Complex to Magnitude-Angle8/1 -> Output5/6
  Data Type Conversion9/1 -> Complex to Magnitude-Angle9/1
  Complex to Magnitude-Angle9/1 -> Output5/7
  Data Type Conversion10/1 -> Complex to Magnitude-Angle10/1
  Complex to Magnitude-Angle10/1 -> Output5/8
  win2/1(cpg_win1) -> Fanout2/1, Data Type Conversion3/1
  win2/2(cpg_win2) -> Fanout3/1, Data Type Conversion6/1
  Demux/5 -> win3/1(mag1)
  Demux/6 -> win3/2(mag2)
  Demux/7 -> win4/1(mag1)
  Demux/8 -> win4/2(mag2)
  win3/1(cpg_win1) -> Fanout4/1, Data Type Conversion7/1
  win3/2(cpg_win2) -> Fanout5/1, Data Type Conversion8/1
  win4/1(cpg_win1) -> Fanout6/1, Data Type Conversion9/1
  win4/2(cpg_win2) -> Fanout7/1, Data Type Conversion10/1
  Data Type Conversion12/1 -> Complex to Magnitude-Angle12/1
  Complex to Magnitude-Angle12/1 -> Output1/1
  Data Type Conversion13/1 -> Complex to Magnitude-Angle13/1
  Complex to Magnitude-Angle13/1 -> Output1/2
  Data Type Conversion14/1 -> Complex to Magnitude-Angle14/1
  Complex to Magnitude-Angle14/1 -> Output1/3
  Data Type Conversion11/1 -> Complex to Magnitude-Angle11/1
  Complex to Magnitude-Angle11/1 -> Output1/4
  One1/1 -> Mux1/1, Mux3/1
  Mux3/1 -> ChannelOut/3
  Mux1/1 -> ChannelOut/4
  Fanout/1 -> Add1/1
  Fanout1/1 -> Add1/2
  Fanout8/1 -> Data Type Conversion12/1, Mux3/3
  Fanout8/2 -> Terminator/1
  Fanout/2 -> Terminator1/1
  Fanout1/2 -> Terminator2/1
  Fanout2/2 -> Terminator3/1
  Fanout3/2 -> Terminator4/1
  Fanout4/2 -> Terminator5/1
  Fanout5/2 -> Terminator6/1
  Fanout6/2 -> Terminator7/1
  Fanout7/2 -> Terminator8/1
  Fanout2/1 -> Add2/1
  Fanout3/1 -> Add2/2
  Fanout4/1 -> Add3/1
  Fanout5/1 -> Add3/2
  Fanout6/1 -> Add4/1
  Fanout7/1 -> Add4/2
  Add1/1 -> Fanout9/1
  Add4/1 -> Fanout12/1
  Add3/1 -> Fanout11/1
  Add2/1 -> Fanout10/1
  Fanout9/1 -> Add5/1
  Fanout10/1 -> Add5/2
  Fanout11/1 -> Add6/1
  Fanout12/1 -> Add6/2
  Fanout9/2 -> Terminator9/1
  Fanout10/2 -> Terminator10/1
  Fanout11/2 -> Terminator11/1
  Fanout12/2 -> Terminator12/1
  Add5/1 -> Fanout13/1
  Add6/1 -> Fanout14/1
  Fanout13/1 -> Add7/1
  Fanout14/1 -> Add7/2
  Fanout13/2 -> Terminator13/1
  Fanout14/2 -> Terminator14/1
  Add7/1 -> Fanout8/1
  ChannelIn/3 -> Fanout15/1
  Fanout15/2 -> latch_1L1/1
  Fanout15/1 -> Counter2/1
  ChannelIn/4 -> Fanout16/1
  Fanout16/1 -> Demux/1
  Fanout16/2 -> latch_1L1/2
  ChannelIn/5 -> Fanout17/1
  Fanout17/2 -> SampleDelay/1
  Fanout17/1 -> SampleDelay2/1

== system downlink_4c2t/DUT/BLIND_CFR/CFR1/PeakCan ==
  v : Inport
  c : Inport  Port=2
  d : Inport  Port=3
  sig : Inport  Port=4
  ChannelIn : DSPBAPrim/ChannelIn  primtype=channelin  nInputs=dspba_internal_get_channel_ports(gcb)  nOutputs=dspba_internal_get_channel_ports(gcb)  omode=Inherit via internal rule  otype=sfix(16)  scale=2^-15  rndmethod=Unbiased  factor=1  satmethod=Symmetric  shift_vec=[0 1 2 -1]  value=2  inPortNames=['v'; 'c'; '0'; '1'; '2'; '3'; '4'; '5'; '6'; '7'; '8'; '9'; 'A'; 'B'; 'D'; 'E'; 'F'; 'G'; 'H'; 'I'; 'J'; 'K'; 'L'; 'M'; 'N'; 'O'; 'P'; 'Q'; 'R'; 'S'; 'T'; 'U'; 'W'; 'X'; 'Y'; 'Z']  outPortNames=['v'; 'c'; '0'; '1'; '2'; '3'; '4'; '5'; '6'; '7'; '8'; '9'; 'A'; 'B'; 'D'; 'E'; 'F'; 'G'; 'H'; 'I'; 'J'; 'K'; 'L'; 'M'; 'N'; 'O'; 'P'; 'Q'; 'R'; 'S'; 'T'; 'U'; 'W'; 'X'; 'Y'; 'Z']  dspbaimage=dspba_prim.jpg  text=fprintf('In');  style=Optimised  dataSignals=2  foldingEnabled=off  channels=1  sampleRate=200  packetBeginPresent=off  packetBeginEnabled=off  visibilities=dspba_ChannelInVis(gcb)  latencyCorrection=0  version=20141013
  ChannelOut1 : DSPBAPrim/ChannelOut  primtype=channelout  nInputs=dspba_internal_get_channel_ports(gcb)  nOutputs=dspba_internal_get_channel_ports(gcb)  omode=Inherit via internal rule  otype=sfix(16)  scale=2^-15  rndmethod=Unbiased  factor=1  satmethod=Symmetric  shift_vec=[0 1 2 -1]  value=1  inPortNames=['v'; 'c'; '0'; '1'; '2'; '3'; '4'; '5'; '6'; '7'; '8'; '9'; 'A'; 'B'; 'D'; 'E'; 'F'; 'G'; 'H'; 'I'; 'J'; 'K'; 'L'; 'M'; 'N'; 'O'; 'P'; 'Q'; 'R'; 'S'; 'T'; 'U'; 'W'; 'X'; 'Y'; 'Z']  outPortNames=['v'; 'c'; '0'; '1'; '2'; '3'; '4'; '5'; '6'; '7'; '8'; '9'; 'A'; 'B'; 'D'; 'E'; 'F'; 'G'; 'H'; 'I'; 'J'; 'K'; 'L'; 'M'; 'N'; 'O'; 'P'; 'Q'; 'R'; 'S'; 'T'; 'U'; 'W'; 'X'; 'Y'; 'Z']  dspbaimage=dspba_prim.jpg  text=fprintf('Out%s', AdvDSPBChannelOutDisplay(latency));  style=Optimised  dataSignals=1  foldingEnabled=off  channels=1  sampleRate=200  packetBeginPresent=off  packetBeginEnabled=off  visibilities=dspba_ChannelOutVis(gcb)  latency=12  latencyCorrection=0  version=20141013
  Complex to Magnitude-Angle : ComplexToMagnitudeAngle  Output=Magnitude
  Complex to Magnitude-Angle1 : ComplexToMagnitudeAngle  Output=Magnitude
  Complex to Magnitude-Angle2 : ComplexToMagnitudeAngle  Output=Magnitude
  Complex to Real-Iag1 : ComplexToRealImag
  Complex to Real-Iag2 : ComplexToRealImag
  Const : DSPBAPrim/Const  primtype=const  nInputs=0  nOutputs=1  omode=Inherit via internal rule  otype=sfix(16)  scale=2^-15  rndmethod=Unbiased  factor=1  satmethod=Symmetric  shift_vec=[0 1 2 -1]  value=0  inPortNames=['+'; '+';]  outPortNames=[' ']  dspbaimage=dspba_prim.jpg  text=fprintf('%s', num2str(value));  style=Optimised  visibilities=8 + 1024  floatPrecision=float32_m23  version=20120820
  Convert : DSPBAPrim/Convert  primtype=convert  nInputs=1  nOutputs=1  omode=Specify via dialog  otype=sfix(16)  scale=2^-15  rndmethod=Unbiased  factor=1  satmethod=None  shift_vec=[0 1 2 -1]  value=round([0:255]/17)  inPortNames=[' '; ' ';]  outPortNames=[' '; 'c']  dspbaimage=dspba_prim.jpg  text=fprintf('convert');  style=Optimised  visibilities=8+64+256+2^17  clipdetect=off  floatPrecision=float32_m23  advOptions=[]  version=20130211
  Convert1 : DSPBAPrim/Convert  primtype=convert  nInputs=1  nOutputs=1  omode=Specify via dialog  otype=sfix(16)  scale=2^-15  rndmethod=Unbiased  factor=1  satmethod=None  shift_vec=[0 1 2 -1]  value=round([0:255]/17)  inPortNames=[' '; ' ';]  outPortNames=[' '; 'c']  dspbaimage=dspba_prim.jpg  text=fprintf('convert');  style=Optimised  visibilities=8+64+256+2^17  clipdetect=off  floatPrecision=float32_m23  advOptions=[]  version=20130211
  Data Type Conversion1 : DataTypeConversion  OutDataTypeStr=double
  Data Type Conversion2 : DataTypeConversion  OutDataTypeStr=double
  Data Type Conversion3 : DataTypeConversion  OutDataTypeStr=double
  Mult : DSPBAPrim/Mult  primtype=mult  nInputs=2  nOutputs=1  omode=Inherit via internal rule  otype=sfix(16)  scale=2^-15  rndmethod=Unbiased  factor=1  satmethod=Symmetric  shift_vec=[0 1 2 -1]  value=0  inPortNames=[' '; ' ';]  outPortNames=[' ']  dspbaimage=dspba_prim.jpg  text=fprintf('X');  style=Optimised  visibilities=8+2^18+2^19  floatPrecision=float32_m23  floatRounding=correct  advOptions=[]  version=20130115
  Mult1 : DSPBAPrim/Mult  primtype=mult  nInputs=2  nOutputs=1  omode=Inherit via internal rule  otype=sfix(16)  scale=2^-15  rndmethod=Unbiased  factor=1  satmethod=Symmetric  shift_vec=[0 1 2 -1]  value=0  inPortNames=[' '; ' ';]  outPortNames=[' ']  dspbaimage=dspba_prim.jpg  text=fprintf('X');  style=Optimised  visibilities=8+2^18+2^19  floatPrecision=float32_m23  floatRounding=correct  advOptions=[]  version=20130115
  Mux : DSPBAPrim/Mux  primtype=mux  nInputs=evalAionMaskParam(gcb,'value',1)+1  nOutputs=1  omode=Inherit via internal rule  otype=sfix(16)  scale=2^-15  rndmethod=Unbiased  factor=1  satmethod=Symmetric  shift_vec=[0 1 2 -1]  value=2  inPortNames=['s '; 'd0'; 'd1'; 'd2'; 'd3'; 'd4'; 'd5'; 'd6'; 'd7'; 'd8'; 'd9';]  outPortNames=[' ']  dspbaimage=dspba_prim.jpg  text=fprintf('%s', primtype);  style=Optimised  visibilities=1032  version=20131025
  Mux1 : DSPBAPrim/Mux  primtype=mux  nInputs=evalAionMaskParam(gcb,'value',1)+1  nOutputs=1  omode=Inherit via internal rule  otype=sfix(16)  scale=2^-15  rndmethod=Unbiased  factor=1  satmethod=Symmetric  shift_vec=[0 1 2 -1]  value=2  inPortNames=['s '; 'd0'; 'd1'; 'd2'; 'd3'; 'd4'; 'd5'; 'd6'; 'd7'; 'd8'; 'd9';]  outPortNames=[' ']  dspbaimage=dspba_prim.jpg  text=fprintf('%s', primtype);  style=Optimised  visibilities=1032  version=20131025
  Output1 : Scope  NumInputPorts=5
  Real-Imag to Complex : RealImagToComplex
  RegField : DSPBAModelBus/RegField  reg_name=cfr_Params.BaseAddr + REG.Scaling  reg_rwmode=Read/Write  reg_msb=15  reg_lsb=0  reg_mode=Specify via dialog  reg_type=ufix(16)  reg_scale=2^-14  reg_init=cfr_Params.Scaling  reg_desc=Scaling value  reg_modal=off  reg_desc0=0  reg_desc1=0  reg_desc2=0  reg_desc3=0  reg_desc4=0  reg_desc5=0  reg_desc6=0  reg_desc7=0  reg_addr=1300  SampleTime=1  version=20090407
  RegField1 : DSPBAModelBus/RegField  reg_name=cfr_Params.BaseAddr + REG.Enable  reg_rwmode=Read/Write  reg_msb=0  reg_lsb=0  reg_mode=Specify via dialog  reg_type=ufix(1)  reg_scale=2^0  reg_init=cfr_Params.Enable  reg_desc=Enable CFR  reg_modal=off  reg_desc0=0  reg_desc1=0  reg_desc2=0  reg_desc3=0  reg_desc4=0  reg_desc5=0  reg_desc6=0  reg_desc7=0  reg_addr=1304  SampleTime=1  version=20090407
  Sub1 : DSPBAPrim/Sub  primtype=sub  nInputs=2  nOutputs=1  omode=Inherit via internal rule  otype=sfix(16)  scale=2^-15  rndmethod=Unbiased  factor=1  satmethod=Symmetric  shift_vec=[0 1 2 -1]  value=0  inPortNames=['+'; '-';]  outPortNames=[' ']  dspbaimage=dspba_prim.jpg  text=fprintf('-');  style=Optimised  visibilities=8  floatRounding=correct  advOptions=[]  version=20130115
  Sub2 : DSPBAPrim/Sub  primtype=sub  nInputs=2  nOutputs=1  omode=Inherit via internal rule  otype=sfix(16)  scale=2^-15  rndmethod=Unbiased  factor=1  satmethod=Symmetric  shift_vec=[0 1 2 -1]  value=0  inPortNames=['+'; '-';]  outPortNames=[' ']  dspbaimage=dspba_prim.jpg  text=fprintf('-');  style=Optimised  visibilities=8  floatRounding=correct  advOptions=[]  version=20130115
  SynthesisInfo : DSPBAPrim/SynthesisInfo  primtype=synthinfo  nInputs=0  nOutputs=0  omode=Inherit via internal rule  otype=sfix(16)  scale=2^-15  rndmethod=Truncate  factor=1  satmethod=Symmetric  shift_vec=[0 1 2 -1]  value=99  inPortNames=[' '; ' ';]  outPortNames=[' ']  dspbaimage=dspba_prim.jpg  text=fprintf('Style=%s', style);  style=Scheduled  visibilities=32768  constraintInUse=off  constraintRelation=>  constraintLimit=20  bitAccurate=off  version=20150220
  qv : Outport
  qc : Outport  Port=2
  q : Outport  Port=3
  wires:
  Data Type Conversion1/1 -> Complex to Magnitude-Angle/1
  Complex to Magnitude-Angle/1 -> Output1/3
  ChannelIn/3 -> Data Type Conversion1/1, Complex to Real-Iag2/1
  Data Type Conversion2/1 -> Complex to Magnitude-Angle1/1
  Complex to Magnitude-Angle1/1 -> Output1/4
  Real-Imag to Complex/1 -> Data Type Conversion3/1, ChannelOut1/3
  ChannelIn/1 -> Output1/1, ChannelOut1/1
  ChannelIn/2 -> Output1/2, ChannelOut1/2
  v/1 -> ChannelIn/1
  d/1 -> ChannelIn/3
  c/1 -> ChannelIn/2
  sig/1 -> ChannelIn/4
  ChannelOut1/1 -> qv/1
  ChannelOut1/2 -> qc/1
  ChannelOut1/3 -> q/1
  ChannelIn/4 -> Complex to Real-Iag1/1, Data Type Conversion2/1
  RegField/1 -> Mult1/1, Mult/2
  Mult/1 -> Convert/1
  Mult1/1 -> Convert1/1
  Sub1/1 -> Mult/1
  Sub2/1 -> Mult1/2
  Convert/1 -> Real-Imag to Complex/1
  Convert1/1 -> Real-Imag to Complex/2
  Data Type Conversion3/1 -> Complex to Magnitude-Angle2/1
  Complex to Magnitude-Angle2/1 -> Output1/5
  RegField1/1 -> Mux/1, Mux1/1
  Complex to Real-Iag2/1 -> Mux/3
  Complex to Real-Iag2/2 -> Mux1/3
  Mux/1 -> Sub1/2
  Mux1/1 -> Sub2/2
  Const/1 -> Mux1/2, Mux/2
  Complex to Real-Iag1/1 -> Sub1/1
  Complex to Real-Iag1/2 -> Sub2/1

== system downlink_4c2t/DUT/BLIND_CFR/CFR1/PulseScale ==
  v : Inport
  c : Inport  Port=2
  d : Inport  Port=3
  ChannelIn : DSPBAPrim/ChannelIn  primtype=channelin  nInputs=dspba_internal_get_channel_ports(gcb)  nOutputs=dspba_internal_get_channel_ports(gcb)  omode=Inherit via internal rule  otype=sfix(16)  scale=2^-15  rndmethod=Unbiased  factor=1  satmethod=Symmetric  shift_vec=[0 1 2 -1]  value=1  inPortNames=['v'; 'c'; '0'; '1'; '2'; '3'; '4'; '5'; '6'; '7'; '8'; '9'; 'A'; 'B'; 'D'; 'E'; 'F'; 'G'; 'H'; 'I'; 'J'; 'K'; 'L'; 'M'; 'N'; 'O'; 'P'; 'Q'; 'R'; 'S'; 'T'; 'U'; 'W'; 'X'; 'Y'; 'Z']  outPortNames=['v'; 'c'; '0'; '1'; '2'; '3'; '4'; '5'; '6'; '7'; '8'; '9'; 'A'; 'B'; 'D'; 'E'; 'F'; 'G'; 'H'; 'I'; 'J'; 'K'; 'L'; 'M'; 'N'; 'O'; 'P'; 'Q'; 'R'; 'S'; 'T'; 'U'; 'W'; 'X'; 'Y'; 'Z']  dspbaimage=dspba_prim.jpg  text=fprintf('In');  style=Optimised  dataSignals=1  foldingEnabled=off  channels=1  sampleRate=200  packetBeginPresent=off  packetBeginEnabled=off  visibilities=dspba_ChannelInVis(gcb)  latencyCorrection=0  version=20141013
  ChannelOut : DSPBAPrim/ChannelOut  primtype=channelout  nInputs=dspba_internal_get_channel_ports(gcb)  nOutputs=dspba_internal_get_channel_ports(gcb)  omode=Inherit via internal rule  otype=sfix(16)  scale=2^-15  rndmethod=Unbiased  factor=1  satmethod=Symmetric  shift_vec=[0 1 2 -1]  value=3  inPortNames=['v'; 'c'; '0'; '1'; '2'; '3'; '4'; '5'; '6'; '7'; '8'; '9'; 'A'; 'B'; 'D'; 'E'; 'F'; 'G'; 'H'; 'I'; 'J'; 'K'; 'L'; 'M'; 'N'; 'O'; 'P'; 'Q'; 'R'; 'S'; 'T'; 'U'; 'W'; 'X'; 'Y'; 'Z']  outPortNames=['v'; 'c'; '0'; '1'; '2'; '3'; '4'; '5'; '6'; '7'; '8'; '9'; 'A'; 'B'; 'D'; 'E'; 'F'; 'G'; 'H'; 'I'; 'J'; 'K'; 'L'; 'M'; 'N'; 'O'; 'P'; 'Q'; 'R'; 'S'; 'T'; 'U'; 'W'; 'X'; 'Y'; 'Z']  dspbaimage=dspba_prim.jpg  text=fprintf('Out%s', AdvDSPBChannelOutDisplay(latency));  style=Optimised  dataSignals=3  foldingEnabled=off  channels=1  sampleRate=200  packetBeginPresent=off  packetBeginEnabled=off  visibilities=dspba_ChannelOutVis(gcb)  latency=30  latencyCorrection=0  version=20141013
  ScalFact : Subsystem
  SynthesisInfo : DSPBAPrim/SynthesisInfo  primtype=synthinfo  nInputs=0  nOutputs=0  omode=Inherit via internal rule  otype=sfix(16)  scale=2^-15  rndmethod=Truncate  factor=1  satmethod=Symmetric  shift_vec=[0 1 2 -1]  value=99  inPortNames=[' '; ' ';]  outPortNames=[' ']  dspbaimage=dspba_prim.jpg  text=fprintf('Style=%s', style);  style=Scheduled  visibilities=32768  constraintInUse=off  constraintRelation=>  constraintLimit=50  bitAccurate=off  version=20150220
  qv : Outport
  qc : Outport  Port=2
  Out_c : Outport  Port=3
  count_o : Outport  Port=4
  sig_i : Outport  Port=5
  wires:
  v/1 -> ChannelIn/1
  c/1 -> ChannelIn/2
  ScalFact/1(qv) -> ChannelOut/1
  ScalFact/2(qc) -> ChannelOut/2
  ScalFact/3(Out_c) -> ChannelOut/3
  d/1 -> ChannelIn/3
  ChannelIn/1 -> ScalFact/1(v)
  ChannelIn/2 -> ScalFact/2(c)
  ChannelIn/3 -> ScalFact/3(d), ChannelOut/5
  ChannelOut/1 -> qv/1
  ChannelOut/2 -> qc/1
  ChannelOut/3 -> Out_c/1
  ScalFact/4(count_o) -> ChannelOut/4
  ChannelOut/4 -> count_o/1
  ChannelOut/5 -> sig_i/1
